simulink model "HEV_Simu_V1_1c"  (R2018b)
settings: configuration reference "Config_Plant" (kept outside this file)
PreLoadFcn:
  | HevSimuVccWs_V1_PreLoad
  | %プラントモデルのコールバック・プリロード関数のバス定義
  | HEVPlant_Ptbs_V1_BusInfo
  | Engine_MapMdl_Ptbs_V1_BusInfo
  | Motor_MapMdl_Ptbs_V1_BusInfo
StartFcn:
  | tic
StopFcn:
  | toc
  | disp(['実時間の' num2str(max(tout)/toc) '倍速'])
libraries: CAN_Lib_V1 x4, simulink x2
settings Model: Creator=E00026  LastModifiedBy=E00026
settings ConfigSetRef: SourceLocation=Base Workspace

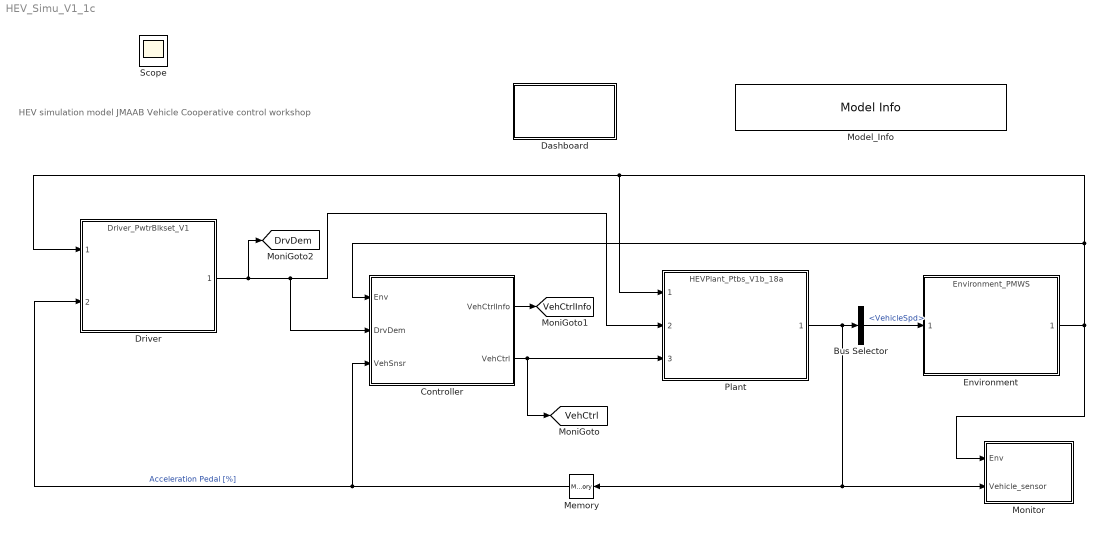
== system HEV_Simu_V1_1c ==
  note: HEV simulation model
      | JMAAB Vehicle Cooperative control workshop
  Bus Selector : BusSelector  OutputSignals=Brake_sensor.VehicleSpd
  Controller : Subsystem  TreatAsAtomicUnit=on  VariantControl=VarObj_CtrlStruct_CAN_VNT_Level_2
  Dashboard : Subsystem
  Driver : ModelReference  ModelNameDialog=Driver_PwtrBlkset_V1.slx  SimulationMode=Normal  ModelReferenceVersion=1.1303
  Environment : ModelReference  ModelNameDialog=Environment_PMWS.slx  SimulationMode=Normal  ModelReferenceVersion=1.1287
  Memory : Memory
  Model_Info : simulink/Model-Wide Utilities/Model Info  Frame=on  DisplayStringWithTags=|  HorizontalTextAlignment=Left  LeftAlignmentValue=0.02
      | Version  %<ModelVersion>
      | LastModifided by %<LastModifiedBy>  Date %<LastModificationDate>
      | Description  %<Description>
  Monitor : Subsystem
  Plant : ModelReference  ModelNameDialog=HEVPlant_Ptbs_V1b_18a.slx  ModelReferenceVersion=1.44
  Scope : Scope
  tag scope: DrvDem=global, VehCtrl=global, VehCtrlInfo=global
  wires:
  Environment/1 -> Controller/1(Env), Plant/1, Driver/1, Monitor/1(Env)
  Controller/1(VehCtrlInfo) -> [VehCtrlInfo]
  Plant/1 -> Monitor/2(Vehicle_sensor), Memory/1, Bus Selector/1
  Driver/1 -> Controller/2(DrvDem), Plant/2, [DrvDem]
  Memory/1 -> Controller/3(VehSnsr), Driver/2  "Acceleration Pedal [%]"
  Controller/2(VehCtrl) -> Plant/3, [VehCtrl]
  Bus Selector/1 -> Environment/1  "<VehicleSpd>"

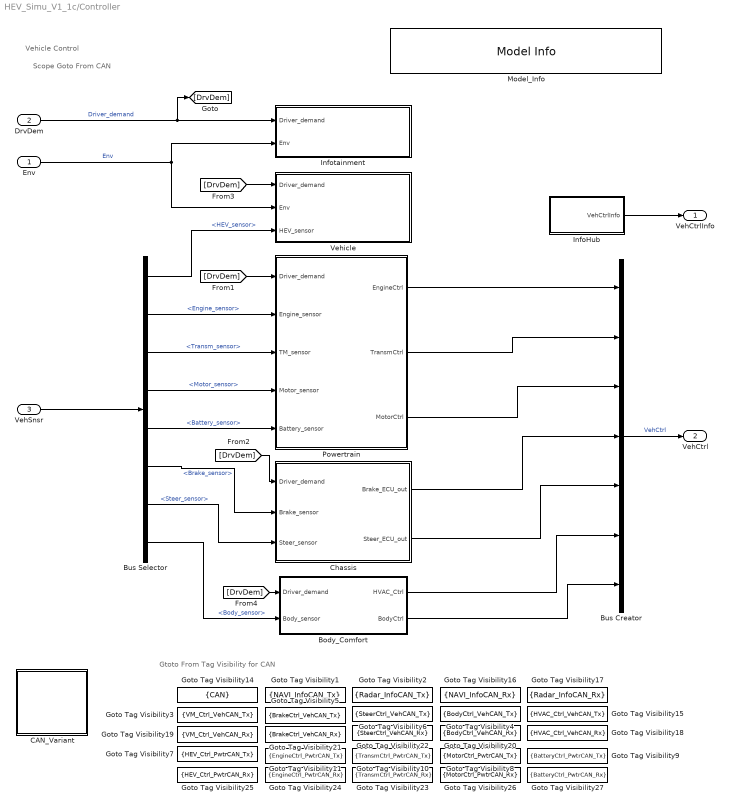
== system HEV_Simu_V1_1c/Controller ==
  note: Vehicle Control
  note: Gtoto From Tag Visibility for CAN
  note: Scope Goto From CAN
  Env : Inport  OutDataTypeStr=Bus: Environment_Bus
      settings: AttributesFormatString=<%<OutDataTypeStr>>
  DrvDem : Inport  Port=2  OutDataTypeStr=Bus: Driver_demand_Bus
      settings: AttributesFormatString=%<OutDataTypeStr>
  VehSnsr : Inport  Port=3  OutDataTypeStr=Bus: Vehicle_sensor_Bus
      settings: AttributesFormatString=<%<OutDataTypeStr>>
  Body_Comfort : Subsystem
  Bus Creator : BusCreator  Inputs=7  OutDataTypeStr=Bus: Ctrl_intg_Bus
      settings: AttributesFormatString=%<OutDataTypeStr>
  Bus Selector : BusSelector  OutputSignals=HEV_sensor,Engine_sensor,Transm_sensor,Motor_sensor,Battery_sensor,Brake_sensor,Steer_sensor,Body_sensor
  CAN_Variant : Subsystem  Variant=on
  Chassis : Subsystem
  Goto Tag Visibility1 : GotoTagVisibility  GotoTag=NAVI_InfoCAN_Tx
  Goto Tag Visibility10 : GotoTagVisibility  GotoTag=TransmCtrl_PwtrCAN_Tx
  Goto Tag Visibility11 : GotoTagVisibility  GotoTag=EngineCtrl_PwtrCAN_Tx
  Goto Tag Visibility14 : GotoTagVisibility  GotoTag=CAN
  Goto Tag Visibility15 : GotoTagVisibility  GotoTag=HVAC_Ctrl_VehCAN_Tx
  Goto Tag Visibility16 : GotoTagVisibility  GotoTag=NAVI_InfoCAN_Rx
  Goto Tag Visibility17 : GotoTagVisibility  GotoTag=Radar_InfoCAN_Rx
  Goto Tag Visibility18 : GotoTagVisibility  GotoTag=HVAC_Ctrl_VehCAN_Rx
  Goto Tag Visibility19 : GotoTagVisibility  GotoTag=VM_Ctrl_VehCAN_Rx
  Goto Tag Visibility2 : GotoTagVisibility  GotoTag=Radar_InfoCAN_Tx
  Goto Tag Visibility20 : GotoTagVisibility  GotoTag=BodyCtrl_VehCAN_Rx
  Goto Tag Visibility21 : GotoTagVisibility  GotoTag=BrakeCtrl_VehCAN_Rx
  Goto Tag Visibility22 : GotoTagVisibility  GotoTag=SteerCtrl_VehCAN_Rx
  Goto Tag Visibility23 : GotoTagVisibility  GotoTag=TransmCtrl_PwtrCAN_Rx
  Goto Tag Visibility24 : GotoTagVisibility  GotoTag=EngineCtrl_PwtrCAN_Rx
  Goto Tag Visibility25 : GotoTagVisibility  GotoTag=HEV_Ctrl_PwtrCAN_Rx
  Goto Tag Visibility26 : GotoTagVisibility  GotoTag=MotorCtrl_PwtrCAN_Rx
  Goto Tag Visibility27 : GotoTagVisibility  GotoTag=BatteryCtrl_PwtrCAN_Rx
  Goto Tag Visibility3 : GotoTagVisibility  GotoTag=VM_Ctrl_VehCAN_Tx
  Goto Tag Visibility4 : GotoTagVisibility  GotoTag=BodyCtrl_VehCAN_Tx
  Goto Tag Visibility5 : GotoTagVisibility  GotoTag=BrakeCtrl_VehCAN_Tx
  Goto Tag Visibility6 : GotoTagVisibility  GotoTag=SteerCtrl_VehCAN_Tx
  Goto Tag Visibility7 : GotoTagVisibility  GotoTag=HEV_Ctrl_PwtrCAN_Tx
  Goto Tag Visibility8 : GotoTagVisibility  GotoTag=MotorCtrl_PwtrCAN_Tx
  Goto Tag Visibility9 : GotoTagVisibility  GotoTag=BatteryCtrl_PwtrCAN_Tx
  InfoHub : Subsystem
  Infotainment : Subsystem
  Model_Info : simulink/Model-Wide Utilities/Model Info  Frame=on  DisplayStringWithTags=|  HorizontalTextAlignment=Left  LeftAlignmentValue=0.02
      | Version  %<ModelVersion>
      | LastModifided by %<LastModifiedBy>  Date %<LastModificationDate>
      | Description  %<Description>
  Powertrain : Subsystem
  Vehicle : Subsystem
  VehCtrlInfo : Outport  OutDataTypeStr=Bus: IntgCtrl_Info_Bus
      settings: AttributesFormatString=<%<OutDataTypeStr>>
  VehCtrl : Outport  Port=2  OutDataTypeStr=Bus: Ctrl_intg_Bus
      settings: AttributesFormatString=<%<OutDataTypeStr>>
  wires:
  Chassis/2(Steer_ECU_out) -> Bus Creator/5
  Powertrain/3(MotorCtrl) -> Bus Creator/3
  Env/1 -> Infotainment/2(Env), Vehicle/2(Env)  "Env"
  Bus Selector/3 -> Powertrain/3(TM_sensor)  "<Transm_sensor>"
  InfoHub/1(VehCtrlInfo) -> VehCtrlInfo/1
  Powertrain/2(TransmCtrl) -> Bus Creator/2
  Bus Selector/6 -> Chassis/2(Brake_sensor)  "<Brake_sensor>"
  [DrvDem] -> Chassis/1(Driver_demand)
  Bus Selector/2 -> Powertrain/2(Engine_sensor)  "<Engine_sensor>"
  Bus Selector/7 -> Chassis/3(Steer_sensor)  "<Steer_sensor>"
  Body_Comfort/2(BodyCtrl) -> Bus Creator/7
  VehSnsr/1 -> Bus Selector/1
  [DrvDem] -> Body_Comfort/1(Driver_demand)
  Bus Selector/4 -> Powertrain/4(Motor_sensor)  "<Motor_sensor>"
  Bus Selector/8 -> Body_Comfort/2(Body_sensor)  "<Body_sensor>"
  Bus Selector/1 -> Vehicle/3(HEV_sensor)  "<HEV_sensor>"
  Powertrain/1(EngineCtrl) -> Bus Creator/1
  Body_Comfort/1(HVAC_Ctrl) -> Bus Creator/6
  Bus Creator/1 -> VehCtrl/1  "VehCtrl"
  [DrvDem] -> Vehicle/1(Driver_demand)
  Bus Selector/5 -> Powertrain/5(Battery_sensor)  "<Battery_sensor>"
  Chassis/1(Brake_ECU_out) -> Bus Creator/4
  [DrvDem] -> Powertrain/1(Driver_demand)
  DrvDem/1 -> Infotainment/1(Driver_demand), [DrvDem]  "Driver_demand"

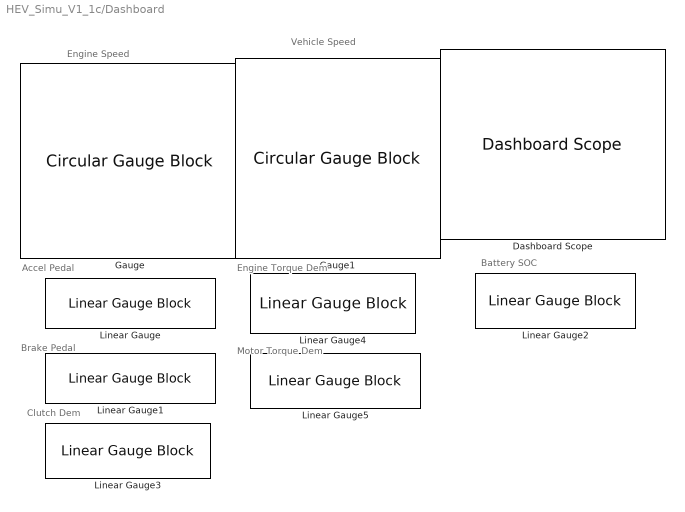
== system HEV_Simu_V1_1c/Dashboard ==
  note: Battery SOC
  note: Brake Pedal
  note: Accel Pedal
  note: Engine Speed
  note: Vehicle Speed
  note: Engine Torque Dem
  note: Clutch Dem
  note: Motor Torque Dem
  Dashboard Scope : DashboardScope  TimeSpan=30  Ymin=0  Ymax=80
  Gauge : CircularGaugeBlock  ScaleMax=4000
  Gauge1 : CircularGaugeBlock  ScaleMax=160  TickInterval=20
  Linear Gauge{,1..2,4} (4 alike) : LinearGaugeBlock
  Linear Gauge3 : LinearGaugeBlock  ScaleMax=1
  Linear Gauge5 : LinearGaugeBlock  ScaleMin=-100

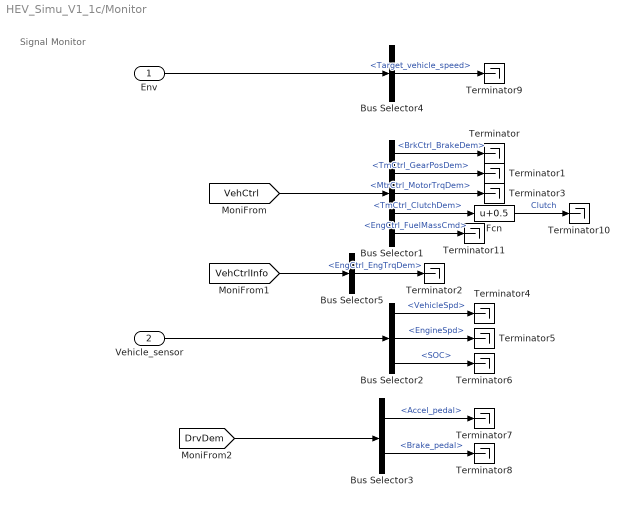
== system HEV_Simu_V1_1c/Monitor ==
  note: Signal Monitor
  Env : Inport
  Vehicle_sensor : Inport  Port=2
  Bus Selector1 : BusSelector  OutputSignals=BrakeCtrl.BrkCtrl_BrakeDem,TransmCtrl.TmCtrl_GearPosDem,MotorCtrl.MtrCtrl_MotorTrqDem,TransmCtrl.TmCtrl_ClutchDem,EngineCtrl.EngCtrl_FuelMassCmd
  Bus Selector2 : BusSelector  OutputSignals=Brake_sensor.VehicleSpd,Engine_sensor.EngineSpd,Battery_sensor.SOC
  Bus Selector3 : BusSelector  OutputSignals=Accel_pedal,Brake_pedal
  Bus Selector4 : BusSelector  OutputSignals=Target_vehicle_speed
  Bus Selector5 : BusSelector  OutputSignals=EngineCtrl_Info.EngCtrl_EngTrqDem
  Fcn : Fcn  Expr=u+0.5
  Terminator{,1..11} (12 alike) : Terminator
  wires:
  [VehCtrl] -> Bus Selector1/1
  Vehicle_sensor/1 -> Bus Selector2/1
  Bus Selector1/2 -> Terminator1/1  "<TmCtrl_GearPosDem>"
  Bus Selector1/3 -> Terminator3/1  "<MtrCtrl_MotorTrqDem>"
  Bus Selector2/1 -> Terminator4/1  "<VehicleSpd>"
  Bus Selector2/2 -> Terminator5/1  "<EngineSpd>"
  Bus Selector2/3 -> Terminator6/1  "<SOC>"
  Bus Selector1/1 -> Terminator/1  "<BrkCtrl_BrakeDem>"
  [DrvDem] -> Bus Selector3/1
  Bus Selector3/1 -> Terminator7/1  "<Accel_pedal>"
  Bus Selector3/2 -> Terminator8/1  "<Brake_pedal>"
  Env/1 -> Bus Selector4/1
  Bus Selector4/1 -> Terminator9/1  "<Target_vehicle_speed>"
  [VehCtrlInfo] -> Bus Selector5/1
  Bus Selector5/1 -> Terminator2/1  "<EngCtrl_EngTrqDem>"
  Bus Selector1/4 -> Fcn/1  "<TmCtrl_ClutchDem>"
  Fcn/1 -> Terminator10/1  "Clutch"
  Bus Selector1/5 -> Terminator11/1  "<EngCtrl_FuelMassCmd>"

== system HEV_Simu_V1_1c/Controller/Body_Comfort ==
  note: Body Control
  Driver_demand : Inport
  Body_sensor : Inport  Port=2
  Body_Control : Subsystem
  HVAC_Control : Subsystem
  HVAC_Ctrl : Outport
  BodyCtrl : Outport  Port=2
  wires:
  HVAC_Control/1(HVAC_Ctrl) -> HVAC_Ctrl/1
  Body_sensor/1 -> Body_Control/2(Body_sensor), HVAC_Control/2(Body_sensor)
  Driver_demand/1 -> Body_Control/1(Driver_demand), HVAC_Control/1(Driver_demand)
  Body_Control/1(BodyCtrl) -> BodyCtrl/1

== system HEV_Simu_V1_1c/Controller/CAN_Variant ==
  note: 1) Add Subsystem or Model blocks as valid variant choices.
      | 2) You cannot connect blocks at this level. At simulation, connectivity is automatically
      | determined, based on the active variant and port name matching.
  Simple_CAN : CAN_Lib_V1/Simple_CAN  SystemSampleTime=-1  VariantControl=VarObj_CanType_Simpl
  Simple_CAN_TW : CAN_Lib_V1/Simple_CAN_TW  SystemSampleTime=-1  VariantControl=VarObj_CanType_Simpl_TW
  VNT_Level1_CAN_TW : CAN_Lib_V1/VNT_Level1_CAN_TW  SystemSampleTime=-1  VariantControl=VarObj_CanType_VNT_Level_1
  VNT_Level_2_CAN : CAN_Lib_V1/VNT_Level_2_CAN  SystemSampleTime=-1  VariantControl=VarObj_CanType_VNT_Level_2

== system HEV_Simu_V1_1c/Controller/Chassis ==
  note: Chassis Control
  Driver_demand : Inport
  Brake_sensor : Inport  Port=2
  Steer_sensor : Inport  Port=3
  Brake_Control : Subsystem
  Steer_Control : Subsystem
  Brake_ECU_out : Outport
  Steer_ECU_out : Outport  Port=2
  wires:
  Steer_sensor/1 -> Steer_Control/2(Steer_sensor)
  Steer_Control/1(SteerCtrl) -> Steer_ECU_out/1
  Brake_sensor/1 -> Brake_Control/2(Brake_sensor)
  Brake_Control/1(BrakeCtrl) -> Brake_ECU_out/1
  Driver_demand/1 -> Steer_Control/1(Driver_demand), Brake_Control/1(Driver_demand)

== system HEV_Simu_V1_1c/Controller/InfoHub ==
  Bus Creator1 : BusCreator  Inputs=2
  VehCtrlInfo : Outport
  wires:
  Bus Creator1/1 -> VehCtrlInfo/1  "VehCtrlInfo"
  [Engine_ECU_Info] -> Bus Creator1/2
  [HEV_ECU_Info] -> Bus Creator1/1

== system HEV_Simu_V1_1c/Controller/Infotainment ==
  note: Infotainment
  Driver_demand : Inport
  Env : Inport  Port=2
  Navigation : Subsystem
  Radar_Detection : Subsystem
  wires:
  Driver_demand/1 -> Navigation/1(Driver_demand), Radar_Detection/1(Driver_demand)
  Env/1 -> Radar_Detection/2(Env), Navigation/2(Env)

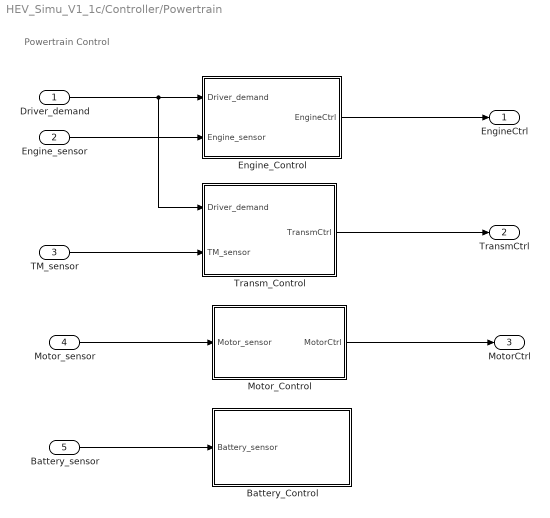
== system HEV_Simu_V1_1c/Controller/Powertrain ==
  note: Powertrain Control
  Driver_demand : Inport
  Engine_sensor : Inport  Port=2
  TM_sensor : Inport  Port=3
  Motor_sensor : Inport  Port=4
  Battery_sensor : Inport  Port=5
  Battery_Control : Subsystem
  Engine_Control : Subsystem
  Motor_Control : Subsystem
  Transm_Control : Subsystem
  EngineCtrl : Outport
  TransmCtrl : Outport  Port=2
  MotorCtrl : Outport  Port=3
  wires:
  TM_sensor/1 -> Transm_Control/2(TM_sensor)
  Transm_Control/1(TransmCtrl) -> TransmCtrl/1
  Engine_sensor/1 -> Engine_Control/2(Engine_sensor)
  Engine_Control/1(EngineCtrl) -> EngineCtrl/1
  Battery_sensor/1 -> Battery_Control/1(Battery_sensor)
  Motor_sensor/1 -> Motor_Control/1(Motor_sensor)
  Motor_Control/1(MotorCtrl) -> MotorCtrl/1
  Driver_demand/1 -> Engine_Control/1(Driver_demand), Transm_Control/1(Driver_demand)

== system HEV_Simu_V1_1c/Controller/Vehicle ==
  note: Vehicle Integrated Control
  Driver_demand : Inport
  Env : Inport  Port=2
  HEV_sensor : Inport  Port=3
  HEV_Control : Subsystem
  Vehicle_Motion_Control : Subsystem
  wires:
  HEV_sensor/1 -> HEV_Control/2(HEV_sensor)
  Driver_demand/1 -> HEV_Control/1(Driver_demand)
  Env/1 -> Vehicle_Motion_Control/1(Env)

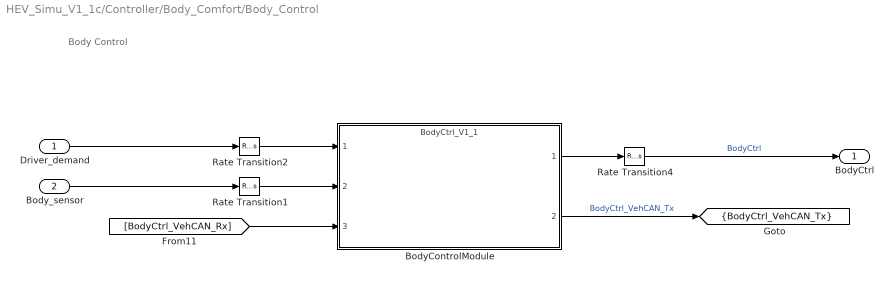
== system HEV_Simu_V1_1c/Controller/Body_Comfort/Body_Control ==
  note: Body Control
  Driver_demand : Inport
  Body_sensor : Inport  Port=2
  BodyControlModule : ModelReference  ModelNameDialog=BodyCtrl_V1_1.slx  SimulationMode=Normal  ModelReferenceVersion=0.1.18
  Rate Transition1 : RateTransition  Deterministic=off
      settings: AttributesFormatString=<Deterministic=%<Deterministic>>
  Rate Transition2 : RateTransition  Deterministic=off
      settings: AttributesFormatString=<Deterministic=%<Deterministic>>
  Rate Transition4 : RateTransition  Deterministic=off
      settings: AttributesFormatString=<Deterministic=%<Deterministic>>
  BodyCtrl : Outport
  tag scope: BodyCtrl_VehCAN_Tx=scoped
  wires:
  Rate Transition1/1 -> BodyControlModule/2
  Body_sensor/1 -> Rate Transition1/1
  Rate Transition4/1 -> BodyCtrl/1  "BodyCtrl"
  BodyControlModule/2 -> [BodyCtrl_VehCAN_Tx]  "BodyCtrl_VehCAN_Tx"
  [BodyCtrl_VehCAN_Rx] -> BodyControlModule/3
  BodyControlModule/1 -> Rate Transition4/1
  Rate Transition2/1 -> BodyControlModule/1
  Driver_demand/1 -> Rate Transition2/1

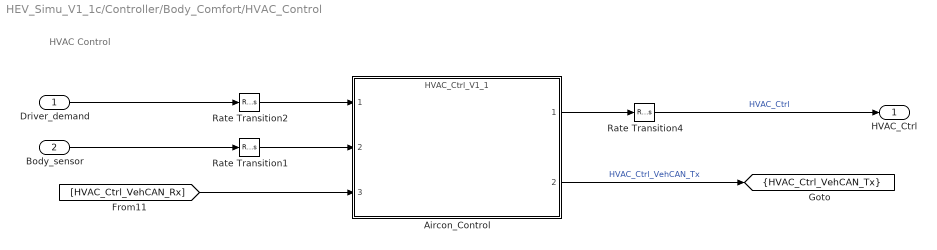
== system HEV_Simu_V1_1c/Controller/Body_Comfort/HVAC_Control ==
  note: HVAC Control
  Driver_demand : Inport
  Body_sensor : Inport  Port=2
  Aircon_Control : ModelReference  ModelNameDialog=HVAC_Ctrl_V1_1.slx  SimulationMode=Normal  ModelReferenceVersion=0.1.27
  Rate Transition1 : RateTransition  Deterministic=off
      settings: AttributesFormatString=<Deterministic=%<Deterministic>>
  Rate Transition2 : RateTransition  Deterministic=off
      settings: AttributesFormatString=<Deterministic=%<Deterministic>>
  Rate Transition4 : RateTransition  Deterministic=off
      settings: AttributesFormatString=<Deterministic=%<Deterministic>>
  HVAC_Ctrl : Outport
  tag scope: HVAC_Ctrl_VehCAN_Tx=scoped
  wires:
  Driver_demand/1 -> Rate Transition2/1
  Rate Transition2/1 -> Aircon_Control/1
  Aircon_Control/1 -> Rate Transition4/1
  [HVAC_Ctrl_VehCAN_Rx] -> Aircon_Control/3
  Aircon_Control/2 -> [HVAC_Ctrl_VehCAN_Tx]  "HVAC_Ctrl_VehCAN_Tx"
  Rate Transition4/1 -> HVAC_Ctrl/1  "HVAC_Ctrl"
  Body_sensor/1 -> Rate Transition1/1
  Rate Transition1/1 -> Aircon_Control/2

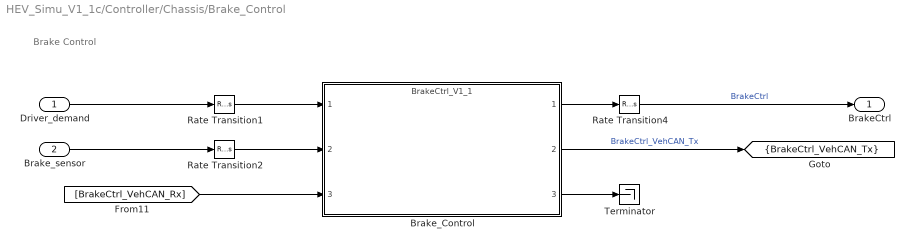
== system HEV_Simu_V1_1c/Controller/Chassis/Brake_Control ==
  note: Brake Control
  Driver_demand : Inport
  Brake_sensor : Inport  Port=2
  Brake_Control : ModelReference  ModelNameDialog=BrakeCtrl_V1_1.slx  SimulationMode=Normal  ModelReferenceVersion=1.0.25
  Rate Transition1 : RateTransition  Deterministic=off
      settings: AttributesFormatString=<Deterministic=%<Deterministic>>
  Rate Transition2 : RateTransition  Deterministic=off
      settings: AttributesFormatString=<Deterministic=%<Deterministic>>
  Rate Transition4 : RateTransition  Deterministic=off
      settings: AttributesFormatString=<Deterministic=%<Deterministic>>
  Terminator : Terminator
  BrakeCtrl : Outport
  tag scope: BrakeCtrl_VehCAN_Tx=scoped
  wires:
  Brake_Control/2 -> [BrakeCtrl_VehCAN_Tx]  "BrakeCtrl_VehCAN_Tx"
  Brake_Control/1 -> Rate Transition4/1
  Rate Transition4/1 -> BrakeCtrl/1  "BrakeCtrl"
  [BrakeCtrl_VehCAN_Rx] -> Brake_Control/3
  Brake_Control/3 -> Terminator/1
  Brake_sensor/1 -> Rate Transition2/1
  Rate Transition1/1 -> Brake_Control/1
  Driver_demand/1 -> Rate Transition1/1
  Rate Transition2/1 -> Brake_Control/2

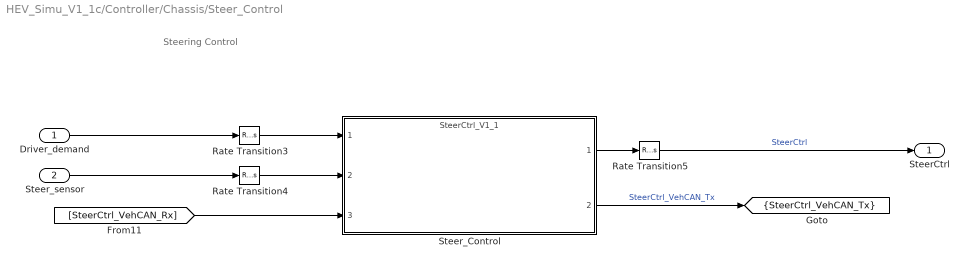
== system HEV_Simu_V1_1c/Controller/Chassis/Steer_Control ==
  note: Steering Control
  Driver_demand : Inport
  Steer_sensor : Inport  Port=2
  Rate Transition3 : RateTransition  Deterministic=off
      settings: AttributesFormatString=<Deterministic=%<Deterministic>>
  Rate Transition4 : RateTransition  Deterministic=off
      settings: AttributesFormatString=<Deterministic=%<Deterministic>>
  Rate Transition5 : RateTransition  Deterministic=off
      settings: AttributesFormatString=<Deterministic=%<Deterministic>>
  Steer_Control : ModelReference  ModelNameDialog=SteerCtrl_V1_1.slx  SimulationMode=Normal  ModelReferenceVersion=0.1.18
  SteerCtrl : Outport
  tag scope: SteerCtrl_VehCAN_Tx=scoped
  wires:
  Steer_Control/2 -> [SteerCtrl_VehCAN_Tx]  "SteerCtrl_VehCAN_Tx"
  Rate Transition5/1 -> SteerCtrl/1  "SteerCtrl"
  Rate Transition3/1 -> Steer_Control/1
  [SteerCtrl_VehCAN_Rx] -> Steer_Control/3
  Steer_sensor/1 -> Rate Transition4/1
  Steer_Control/1 -> Rate Transition5/1
  Driver_demand/1 -> Rate Transition3/1
  Rate Transition4/1 -> Steer_Control/2

== system HEV_Simu_V1_1c/Controller/Infotainment/Navigation ==
  note: Navigation
  Driver_demand : Inport
  Env : Inport  Port=2
  NAVI : ModelReference  ModelNameDialog=NAVI_V1_1.slx  SimulationMode=Normal  ModelReferenceVersion=0.1.19
  Rate Transition1 : RateTransition  Deterministic=off
      settings: AttributesFormatString=<Deterministic=%<Deterministic>>
  Rate Transition4 : RateTransition  Deterministic=off
      settings: AttributesFormatString=<Deterministic=%<Deterministic>>
  tag scope: NAVI_InfoCAN_Tx=scoped
  wires:
  Rate Transition4/1 -> NAVI/2
  Env/1 -> Rate Transition4/1
  NAVI/1 -> [NAVI_InfoCAN_Tx]  "NAVI_InfoCAN_Tx"
  [NAVI_InfoCAN_Rx] -> NAVI/3
  Driver_demand/1 -> Rate Transition1/1
  Rate Transition1/1 -> NAVI/1

== system HEV_Simu_V1_1c/Controller/Infotainment/Radar_Detection ==
  note: Radar Detection
  Driver_demand : Inport
  Env : Inport  Port=2
  Radar_Detection : ModelReference  ModelNameDialog=Radar_V1_1.slx  SimulationMode=Normal  ModelReferenceVersion=0.1.19
  Rate Transition1 : RateTransition  Deterministic=off
      settings: AttributesFormatString=<Deterministic=%<Deterministic>>
  Rate Transition4 : RateTransition  Deterministic=off
      settings: AttributesFormatString=<Deterministic=%<Deterministic>>
  tag scope: Radar_InfoCAN_Tx=scoped
  wires:
  Rate Transition4/1 -> Radar_Detection/1
  Driver_demand/1 -> Rate Transition4/1
  Radar_Detection/1 -> [Radar_InfoCAN_Tx]  "Radar_InfoCAN_Tx"
  [Radar_InfoCAN_Rx] -> Radar_Detection/3
  Env/1 -> Rate Transition1/1
  Rate Transition1/1 -> Radar_Detection/2

== system HEV_Simu_V1_1c/Controller/Powertrain/Battery_Control ==
  note: Battery Control
  Battery_sensor : Inport
  Battery_Control : ModelReference  ModelNameDialog=BatteryCtrl_V1_1.slx  SimulationMode=Normal  ModelReferenceVersion=0.1.24
  Rate Transition1 : RateTransition  Deterministic=off
      settings: AttributesFormatString=<Deterministic=%<Deterministic>>
  tag scope: BatteryCtrl_PwtrCAN_Tx=scoped
  wires:
  Battery_Control/1 -> [BatteryCtrl_PwtrCAN_Tx]  "BatteryCtrl_PwtrCAN_Tx"
  Rate Transition1/1 -> Battery_Control/1
  [BatteryCtrl_PwtrCAN_Rx] -> Battery_Control/2
  Battery_sensor/1 -> Rate Transition1/1

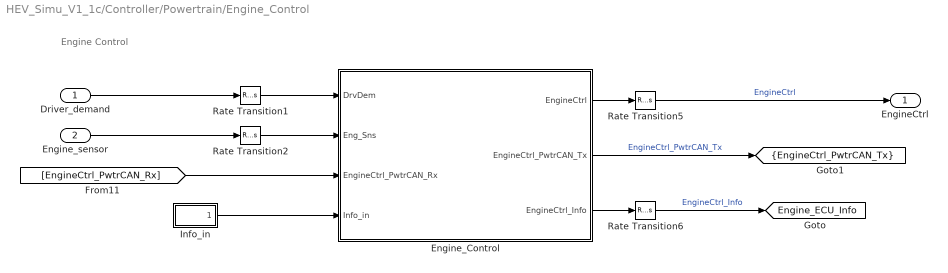
== system HEV_Simu_V1_1c/Controller/Powertrain/Engine_Control ==
  note: Engine Control
  Driver_demand : Inport
  Engine_sensor : Inport  Port=2
  Engine_Control : Subsystem  Variant=on
  Info_in : Subsystem
  Rate Transition{1..2,5..6} (4 alike) : RateTransition  Deterministic=off
      settings: AttributesFormatString=<Deterministic=%<Deterministic>>
  EngineCtrl : Outport
  tag scope: EngineCtrl_PwtrCAN_Tx=scoped, Engine_ECU_Info=global
  wires:
  Engine_Control/3(" EngineCtrl_Info") -> Rate Transition6/1
  Engine_Control/1(" EngineCtrl") -> Rate Transition5/1
  Info_in/1(Info_in) -> Engine_Control/4("Info_in ")
  [EngineCtrl_PwtrCAN_Rx] -> Engine_Control/3(EngineCtrl_PwtrCAN_Rx)
  Rate Transition2/1 -> Engine_Control/2("Eng_Sns ")
  Rate Transition1/1 -> Engine_Control/1("DrvDem ")
  Engine_Control/2(" EngineCtrl_PwtrCAN_Tx") -> [EngineCtrl_PwtrCAN_Tx]  "EngineCtrl_PwtrCAN_Tx"
  Rate Transition6/1 -> [Engine_ECU_Info]  "EngineCtrl_Info"
  Rate Transition5/1 -> EngineCtrl/1  "EngineCtrl"
  Engine_sensor/1 -> Rate Transition2/1
  Driver_demand/1 -> Rate Transition1/1

== system HEV_Simu_V1_1c/Controller/Powertrain/Motor_Control ==
  note: Motor Control
  Motor_sensor : Inport
  Motor_Control : ModelReference  ModelNameDialog=MotorCtrl_V1_1.slx  SimulationMode=Normal  ModelReferenceVersion=1.0.23
  Rate Transition1 : RateTransition  Deterministic=off
      settings: AttributesFormatString=<Deterministic=%<Deterministic>>
  Rate Transition3 : RateTransition  Deterministic=off
      settings: AttributesFormatString=<Deterministic=%<Deterministic>>
  Terminator : Terminator
  MotorCtrl : Outport
  tag scope: MotorCtrl_PwtrCAN_Tx=scoped
  wires:
  Motor_Control/2 -> [MotorCtrl_PwtrCAN_Tx]  "MotorCtrl_PwtrCAN_Tx"
  Motor_Control/1 -> Rate Transition3/1
  Rate Transition3/1 -> MotorCtrl/1  "MotorCtrl"
  Motor_Control/3 -> Terminator/1
  Motor_sensor/1 -> Rate Transition1/1
  [MotorCtrl_PwtrCAN_Rx] -> Motor_Control/2
  Rate Transition1/1 -> Motor_Control/1

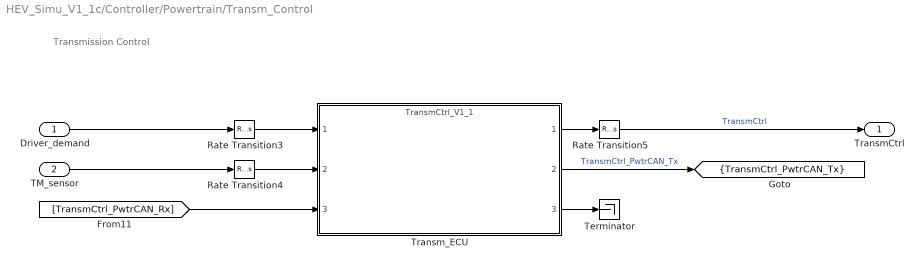
== system HEV_Simu_V1_1c/Controller/Powertrain/Transm_Control ==
  note: Transmission Control
  Driver_demand : Inport
  TM_sensor : Inport  Port=2
  Rate Transition3 : RateTransition  Deterministic=off
      settings: AttributesFormatString=<Deterministic=%<Deterministic>>
  Rate Transition4 : RateTransition  Deterministic=off
      settings: AttributesFormatString=<Deterministic=%<Deterministic>>
  Rate Transition5 : RateTransition  Deterministic=off
      settings: AttributesFormatString=<Deterministic=%<Deterministic>>
  Terminator : Terminator
  Transm_ECU : ModelReference  ModelNameDialog=TransmCtrl_V1_1.slx  SimulationMode=Normal  ModelReferenceVersion=1.0.43
  TransmCtrl : Outport
  tag scope: TransmCtrl_PwtrCAN_Tx=scoped
  wires:
  Transm_ECU/2 -> [TransmCtrl_PwtrCAN_Tx]  "TransmCtrl_PwtrCAN_Tx"
  Transm_ECU/1 -> Rate Transition5/1
  Rate Transition5/1 -> TransmCtrl/1  "TransmCtrl"
  Rate Transition3/1 -> Transm_ECU/1
  [TransmCtrl_PwtrCAN_Rx] -> Transm_ECU/3
  TM_sensor/1 -> Rate Transition4/1
  Driver_demand/1 -> Rate Transition3/1
  Transm_ECU/3 -> Terminator/1
  Rate Transition4/1 -> Transm_ECU/2

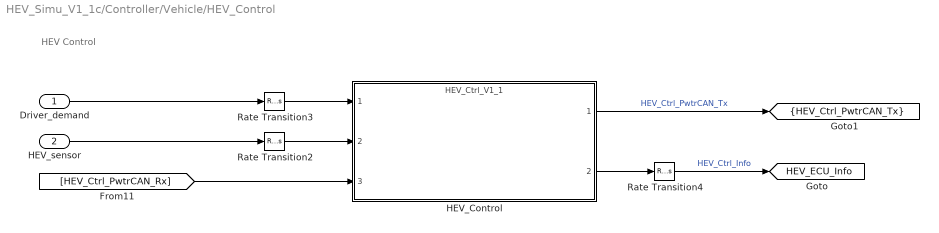
== system HEV_Simu_V1_1c/Controller/Vehicle/HEV_Control ==
  note: HEV Control
  Driver_demand : Inport
  HEV_sensor : Inport  Port=2
  HEV_Control : ModelReference  ModelNameDialog=HEV_Ctrl_V1_1.slx  SimulationMode=Normal  ModelReferenceVersion=1.0.64
  Rate Transition2 : RateTransition  Deterministic=off
      settings: AttributesFormatString=<Deterministic=%<Deterministic>>
  Rate Transition3 : RateTransition  Deterministic=off
      settings: AttributesFormatString=<Deterministic=%<Deterministic>>
  Rate Transition4 : RateTransition  Deterministic=off
      settings: AttributesFormatString=<Deterministic=%<Deterministic>>
  tag scope: HEV_Ctrl_PwtrCAN_Tx=scoped, HEV_ECU_Info=global
  wires:
  Rate Transition3/1 -> HEV_Control/1
  HEV_Control/1 -> [HEV_Ctrl_PwtrCAN_Tx]  "HEV_Ctrl_PwtrCAN_Tx"
  Rate Transition4/1 -> [HEV_ECU_Info]  "HEV_Ctrl_Info"
  HEV_Control/2 -> Rate Transition4/1
  Rate Transition2/1 -> HEV_Control/2
  HEV_sensor/1 -> Rate Transition2/1
  [HEV_Ctrl_PwtrCAN_Rx] -> HEV_Control/3
  Driver_demand/1 -> Rate Transition3/1

== system HEV_Simu_V1_1c/Controller/Vehicle/Vehicle_Motion_Control ==
  note: Vehicle Motion Control
  Env : Inport
  Rate Transition1 : RateTransition  Deterministic=off
      settings: AttributesFormatString=<Deterministic=%<Deterministic>>
  Vehicle_Motion_Control : ModelReference  ModelNameDialog=VM_Ctrl_V1_1.slx  SimulationMode=Normal  ModelReferenceVersion=0.1.28
  tag scope: VM_Ctrl_VehCAN_Tx=scoped
  wires:
  [VM_Ctrl_VehCAN_Rx] -> Vehicle_Motion_Control/2
  Env/1 -> Rate Transition1/1
  Rate Transition1/1 -> Vehicle_Motion_Control/1
  Vehicle_Motion_Control/1 -> [VM_Ctrl_VehCAN_Tx]  "VM_Ctrl_VehCAN_Tx"

== system HEV_Simu_V1_1c/Controller/Powertrain/Engine_Control/Engine_Control ==
  "DrvDem " : Inport
  "Eng_Sns " : Inport  Port=2
  EngineCtrl_PwtrCAN_Rx : Inport  Port=3
  "Info_in " : Inport  Port=4
  EngineCtrl_V1.slx : ModelReference  ModelNameDialog=EngineCtrl_V1_1.slx  SimulationMode=Normal  VariantControl=VarObj_EngEcu_Simple  ModelReferenceVersion=1.0.27
  EngineCtrl_V2.slx : ModelReference  ModelNameDialog=EngineCtrl_V2.slx  SimulationMode=Normal  VariantControl=VarObj_EngEcu_Medium  ModelReferenceVersion=1.0.8
  " EngineCtrl" : Outport
  " EngineCtrl_PwtrCAN_Tx" : Outport  Port=2
  " EngineCtrl_Info" : Outport  Port=3

== system HEV_Simu_V1_1c/Controller/Powertrain/Engine_Control/Info_in ==
  Bus Creator1 : BusCreator  Inputs=1
  Constant : Constant
  Info_in : Outport
  wires:
  Bus Creator1/1 -> Info_in/1  "Info_in"
  Constant/1 -> Bus Creator1/1  "dummy"
